simulink model "osc_2r"  (R2018a)
settings: Solver=VariableStepAuto  StartTime=0.0  StopTime=10.0  RelTol=1e-3
settings Model: Creator=klukomski  LastModifiedBy=klukomski

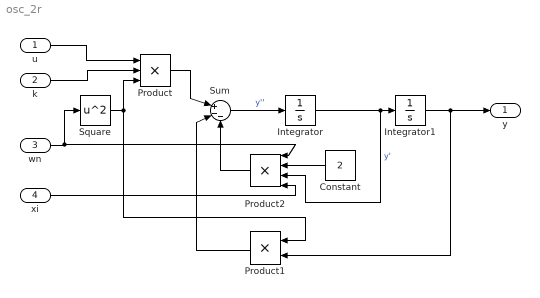
== system osc_2r ==
  "u " : Inport
  k : Inport  Port=2
  wn : Inport  Port=3
  xi : Inport  Port=4
  Constant : Constant  Value=2
  Integrator : Integrator
  Integrator1 : Integrator
  Product : Product  Inputs=3
  Product1 : Product
  Product2 : Product  Inputs=4
  Square : Math  Operator=square  SaturateOnIntegerOverflow=on
  Sum : Sum  Inputs=|+--
  y : Outport
  wires:
  Integrator1/1 -> Product1/2, y/1
  Sum/1 -> Integrator/1  "y''"
  Integrator/1 -> Integrator1/1, Product2/3  "y'"
  "u "/1 -> Product/1
  k/1 -> Product/2
  wn/1 -> Product2/1, Square/1
  Square/1 -> Product1/1, Product/3
  Product/1 -> Sum/1
  xi/1 -> Product2/4
  Constant/1 -> Product2/2
  Product2/1 -> Sum/3
  Product1/1 -> Sum/2
